simulink model "MPPT_PnO_Demo_Block_Implementation"  (R2020a)
settings: Solver=ode23tb  StartTime=0.0  StopTime=10  RelTol=1e-3
libraries: powerlib x4, powerlib_meascontrol x1, re_lib x1
settings Model: Creator=Rodney Tan  LastModifiedBy=Rodney Tan
settings SolverCC: ZeroCrossAlgorithm=Adaptive
settings DataIOCC: ReturnWorkspaceOutputs=off
settings DebuggingCC: MaxConsecutiveZCsMsg=none  ArithmeticOperatorsInVariantConditions=warning
settings SFSimCC: SimUseLocalCustomCode=off  CustomCodeUndefinedFunction=UseInterfaceOnly
settings RTWCC: RTWUseLocalCustomCode=off

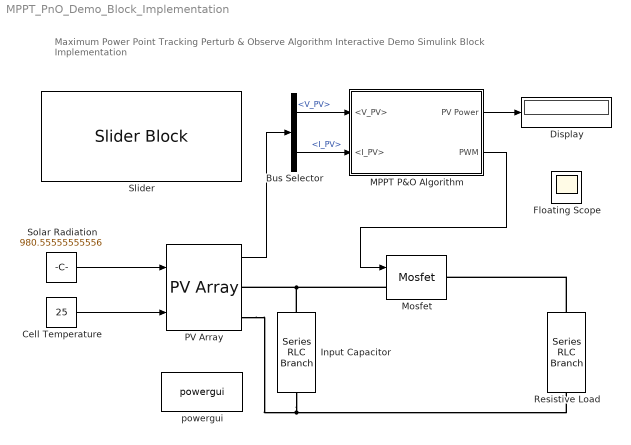
== system MPPT_PnO_Demo_Block_Implementation ==
  note: Maximum Power Point Tracking Perturb & Observe Algorithm Interactive Demo
      | Simulink Block Implementation
  Bus Selector : BusSelector  OutputSignals=V_PV,I_PV
  Cell Temperature : Constant  Value=25
  Display : Display
  Floating Scope : Scope
      settings: Floating=on
  Input Capacitor : powerlib/Elements/Series RLC Branch  LConnTagsString=__new0  RConnTagsString=__new0  BranchType=C  Resistance=10  Inductance=1e-3  SetiL0=off  InitialCurrent=0  Capacitance=1000e-6  Setx0=off  InitialVoltage=0  Measurements=None
  MPPT P&O Algorithm : Subsystem  mask(MPPT Perturb and Observe Algorithm Block){Fsw=1000, StepSize=1e-6}
      mask prompts: Fsw "PWM Switching frequency (Hz):"; StepSize "PWM Duty Cycle (delta) Step Size"
      mask help:
      | MPPT Perturb & Observe Algorithm Block
      | Developed by Rodney Tan (PhD)
      | Version 1.00 Sep 2019
      |
      | This block perform photovoltaic panel Maximum Power Point Tracking based on Perturb & Observe algorithm.
      | This MPPT P&O method is implemented using basic Simulink block only.
      | This MPPT block take in Voltage and Current from photovoltaic panel and output PWM switching signal to drive the DC converter
      mask Help:
      | <b><u>Block Setting</u></b>
      | <b>PWM Switching Frequency (Hz)</b>
      | Specify the PWM switching frequency in Hz.
      | 
      | <b>PWM Duty Cycle Step Size</b>
      | Specify the PWM duty cycle (delta) step size. Default value is 1e-6.
      mask TypeOptions Fsw:
      | PWM Generator
      | (DC-DC)/Fsw
  Mosfet : powerlib/Power Electronics/Mosfet  Ron=0.1  Lon=0  Rd=0.01  Vfd=0  IC=0  Rs=1e5  Cs=inf  Measurements=off
  PV Array : re_lib/Solar/PV Array  Npar=1  Nser=4  PlotType=array @ 1000 W/m2 & specified temperatures  S_vec="[ 1000  500  100 ]"  Temp_C_vec="[ 45 25  ]"  ModuleName=1Soltech 1STH-250-WH  PlotWhenSelected=off  Pm=250.205  Ncell=60  Voc=37.3  Isc=8.66  Vm=30.7  Im=8.15  beta_Voc_pc=-0.36901  alpha_Isc_pc=0.086998  beta_Voc=-0.13764  alpha_Isc=0.007534  IL=8.7106  I0=4.1601e-10  nI=1.019  Rsh=224.1886  Rs=0.23724  RobustModel=off  RobustCellTemperature=25  BAL=on  Tc=1e-6  Tfilter=5e-5
  Resistive Load : powerlib/Elements/Series RLC Branch  LConnTagsString=__new0  RConnTagsString=__new0  BranchType=R  Resistance=5  Inductance=1e-3  SetiL0=off  InitialCurrent=0  Capacitance=1e-6  Setx0=off  InitialVoltage=0  Measurements=None
  Slider : SliderBlock  ScaleMax=1000
  Solar Radiation : Constant  Value=980.55555555556
  powergui : powerlib/powergui  Priority=1  SimulationMode=Discrete  SampleTime=1e-5  frequency=60  Iterations=50  frequencyindice=0  Pbase=100e6  ErrMax=1e-4  UnitsV=kV  UnitsW=MW  buscounter=0  FunctionMessages=off  echomessages=off  EnableUseOfTLC=off  CurrentSourceSwitches=off  DisableSnubberDevices=off  DisableRonSwitches=off  DisableVfSwitches=off  DisplayEquations=off  AutomaticDiscreteSolvers=off  SolverType=Tustin/Backward Euler (TBE)  Interpol=off  ExternalGateDelay=off  methode=off  Ts=100  x0status=blocks  SPID=off  SwTol=0  HookPort=off  NonlinearTolerance=1e-4  nMaxIteration=100  ContinueOnMaxIteration=off  RestoreLinks=warning  ResistiveCurrentMeasurement=off  Frange=[0:2:500]  Ylog=off  Xlog=on  ShowGrid=off  save=off  variable=ZData  structure=0  ZoomFFT=off  StartTime=0.0  cycles=1  DisplayStyle=1  fundamental=60  FreqAxis=off  MaxFrequency=1000  frequencyindicesteady=1  RmsSteady=1  display=off
  wires:
  PV Array/1 -> Bus Selector/1
  Cell Temperature/1 -> PV Array/2
  MPPT P&O Algorithm/2(PWM) -> Mosfet/1
  Bus Selector/1 -> MPPT P&O Algorithm/1(<V_PV>)  "<V_PV>"
  Bus Selector/2 -> MPPT P&O Algorithm/2(<I_PV>)  "<I_PV>"
  MPPT P&O Algorithm/1(PV Power) -> Display/1
  Solar Radiation/1 -> PV Array/1
  connections:
  PV Array/RConn2 -- Resistive Load/RConn1 -- Input Capacitor/RConn1
  Mosfet/LConn1 -- Input Capacitor/LConn1 -- PV Array/RConn1
  Resistive Load/LConn1 -- Mosfet/RConn1

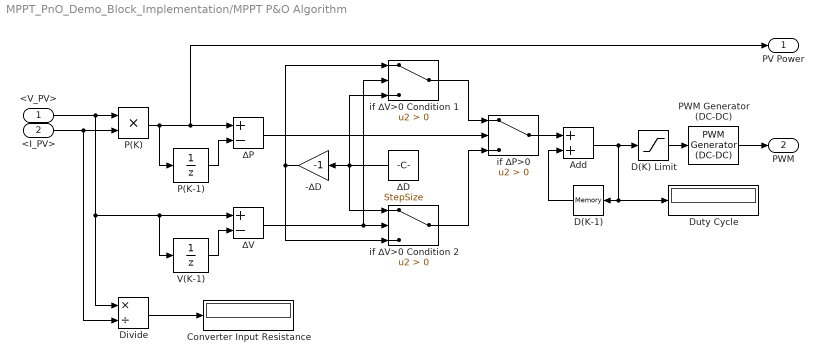
== system MPPT_PnO_Demo_Block_Implementation/MPPT P&O Algorithm ==
  <V_PV> : Inport
  <I_PV> : Inport  Port=2
  -∆D : Gain  Gain=-1
  Add : Sum
  Converter Input Resistance : Display
  D(K) Limit : Saturate  UpperLimit=1  LowerLimit=0
  D(K-1) : Memory  InitialCondition=0.5  InheritSampleTime=on
  Divide : Product  Inputs=*/
  Duty Cycle : Display
  P(K) : Product
  P(K-1) : UnitDelay  SampleTime=-1  HasFrameUpgradeWarning=on
  PWM Generator (DC-DC) : powerlib_meascontrol/Pulse & Signal Generators/PWM Generator (DC-DC)  Fsw=Fsw  Ts=0
  V(K-1) : UnitDelay  SampleTime=-1  HasFrameUpgradeWarning=on
  if ∆P>0 : Switch  Criteria=u2 > Threshold
  if ∆V>0 Condition 1 : Switch  Criteria=u2 > Threshold
  if ∆V>0 Condition 2 : Switch  Criteria=u2 > Threshold
  ∆D : Constant  Value=StepSize
  ∆P : Sum  Inputs=+-
  ∆V : Sum  Inputs=+-
  PV Power : Outport  VectorParamsAs1DForOutWhenUnconnected=off
  PWM : Outport  Port=2  VectorParamsAs1DForOutWhenUnconnected=off
  wires:
  P(K)/1 -> ∆P/1, PV Power/1, P(K-1)/1
  <I_PV>/1 -> P(K)/2, Divide/2
  if ∆P>0/1 -> Add/1
  if ∆V>0 Condition 1/1 -> if ∆P>0/1
  ∆P/1 -> if ∆P>0/2
  P(K-1)/1 -> ∆P/2
  V(K-1)/1 -> ∆V/2
  ∆V/1 -> if ∆V>0 Condition 2/2, if ∆V>0 Condition 1/2
  <V_PV>/1 -> Divide/1, ∆V/1, V(K-1)/1, P(K)/1
  Add/1 -> D(K) Limit/1, Duty Cycle/1, D(K-1)/1
  if ∆V>0 Condition 2/1 -> if ∆P>0/3
  D(K-1)/1 -> Add/2
  ∆D/1 -> if ∆V>0 Condition 2/1, -∆D/1, if ∆V>0 Condition 1/3
  -∆D/1 -> if ∆V>0 Condition 2/3, if ∆V>0 Condition 1/1
  PWM Generator (DC-DC)/1 -> PWM/1
  Divide/1 -> Converter Input Resistance/1
  D(K) Limit/1 -> PWM Generator (DC-DC)/1
